simulink model "Tut16_TriggeredSubsystem"  (R2021a)
settings: Solver=FixedStepDiscrete  StartTime=0.0  StopTime=30  FixedStep=1  RelTol=1e-3
settings Model: Creator=cheta  LastModifiedBy=cheta

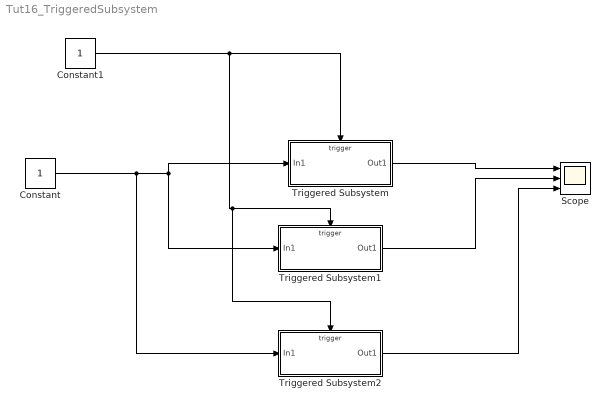
== system Tut16_TriggeredSubsystem ==
  Constant : Constant
  Constant1 : Constant
  Scope : Scope  NumInputPorts=3
  Triggered Subsystem : Subsystem  TreatAsAtomicUnit=on
  Triggered Subsystem1 : Subsystem  TreatAsAtomicUnit=on
  Triggered Subsystem2 : Subsystem  TreatAsAtomicUnit=on
  wires:
  Constant/1 -> Triggered Subsystem2/1(In1), Triggered Subsystem/1(In1), Triggered Subsystem1/1(In1)
  Triggered Subsystem/1(Out1) -> Scope/1
  Constant1/1 -> Triggered Subsystem2/Trigger, Triggered Subsystem1/Trigger, Triggered Subsystem/Trigger
  Triggered Subsystem1/1(Out1) -> Scope/2
  Triggered Subsystem2/1(Out1) -> Scope/3

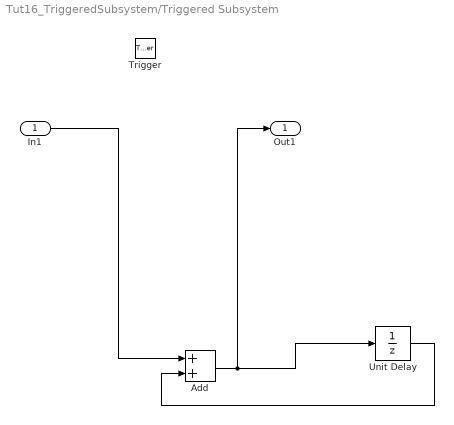
== system Tut16_TriggeredSubsystem/Triggered Subsystem ==
  In1 : Inport
  Trigger : TriggerPort  VariantControl=(inherit)
  Add : Sum
  Unit Delay : UnitDelay  SampleTime=-1  HasFrameUpgradeWarning=on
  Out1 : Outport
  wires:
  In1/1 -> Add/1
  Add/1 -> Out1/1, Unit Delay/1
  Unit Delay/1 -> Add/2

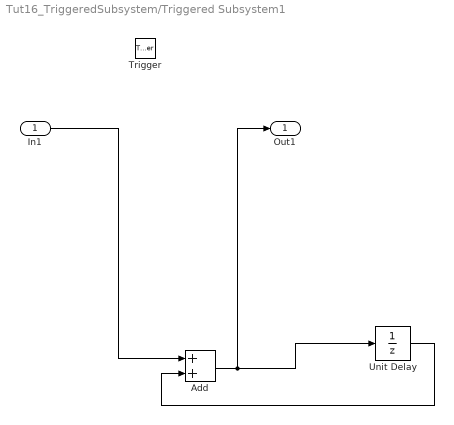
== system Tut16_TriggeredSubsystem/Triggered Subsystem1 ==
  In1 : Inport
  Trigger : TriggerPort  TriggerType=falling  VariantControl=(inherit)
  Add : Sum
  Unit Delay : UnitDelay  SampleTime=-1  HasFrameUpgradeWarning=on
  Out1 : Outport
  wires:
  Unit Delay/1 -> Add/2
  Add/1 -> Unit Delay/1, Out1/1
  In1/1 -> Add/1

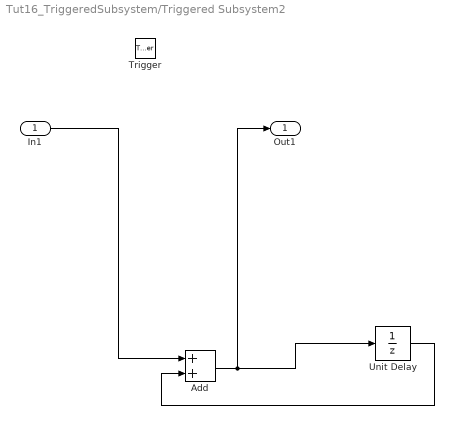
== system Tut16_TriggeredSubsystem/Triggered Subsystem2 ==
  In1 : Inport
  Trigger : TriggerPort  TriggerType=either  VariantControl=(inherit)
  Add : Sum
  Unit Delay : UnitDelay  SampleTime=-1  HasFrameUpgradeWarning=on
  Out1 : Outport
  wires:
  In1/1 -> Add/1
  Add/1 -> Out1/1, Unit Delay/1
  Unit Delay/1 -> Add/2
